simulink library "Lib_General"  (R2023a)
settings: Solver=VariableStepAuto  StartTime=0.0  StopTime=10.0  RelTol=1e-3
settings Model: Creator=62555  LastModifiedBy=62555

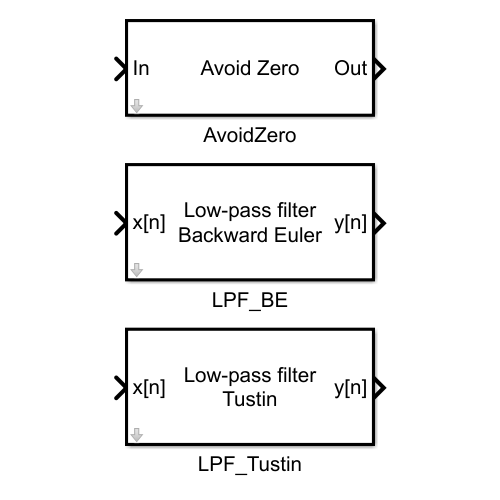
[thumbnail: Simulink's stored preview of the top-level diagram]
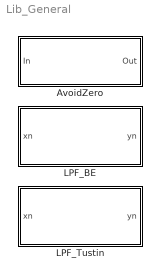
== system Lib_General ==
  AvoidZero : Subsystem  TreatAsAtomicUnit=on  RTWFileName=Lib_General  mask{Min=single(eps)}
      settings: RTWFcnNameOpts=Use subsystem name  RTWFileNameOpts=User specified
      mask Display:
      | disp('Avoid Zero');
      | port_label('input', 1, 'In');
      | port_label('output', 1, 'Out');
  LPF_BE : Subsystem  TreatAsAtomicUnit=on  RTWFileName=Lib_General  mask{fc=1, Ts=1, Initial_condition=0}
      settings: RTWFcnNameOpts=Use subsystem name  RTWFileNameOpts=User specified
      mask Display:
      | disp('Low-pass filter\nBackward Euler');
      | port_label('input', 1, 'x[n]');
      | port_label('output', 1, 'y[n]');
  LPF_Tustin : Subsystem  TreatAsAtomicUnit=on  RTWFileName=Lib_General  mask{fc=1, Ts=1, Initial_condition=0}
      settings: RTWFcnNameOpts=Use subsystem name  RTWFileNameOpts=User specified
      mask Display:
      | disp('Low-pass filter\nTustin');
      | port_label('input', 1, 'x[n]');
      | port_label('output', 1, 'y[n]');

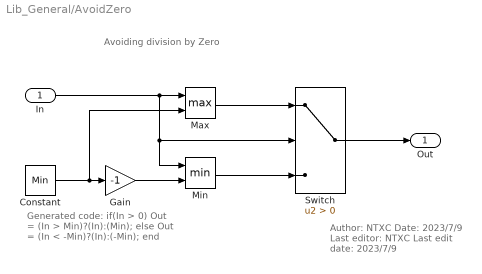
== system Lib_General/AvoidZero ==
  note: Avoiding division by Zero
  note: Generated code:
      |
      | if(In > 0)
      |   Out = (In > Min)?(In):(Min);
      | else
      |   Out = (In < -Min)?(In):(-Min);
      | end
  note: Author: NTXC
      | Date: 2023/7/9
      | Last editor: NTXC
      | Last edit date: 2023/7/9
  In : Inport
  Constant : Constant  Value=Min  OutDataTypeStr=single  SampleTime=-1
  Gain : Gain  Gain=-1
  Max : MinMax  Function=max  Inputs=2
  Min : MinMax  Inputs=2
  Switch : Switch  Criteria=u2 > Threshold  SaturateOnIntegerOverflow=off  InputSameDT=off
  Out : Outport
  wires:
  In/1 -> Min/1, Switch/2, Max/1
  Max/1 -> Switch/1
  Gain/1 -> Min/2
  Min/1 -> Switch/3
  Constant/1 -> Max/2, Gain/1
  Switch/1 -> Out/1

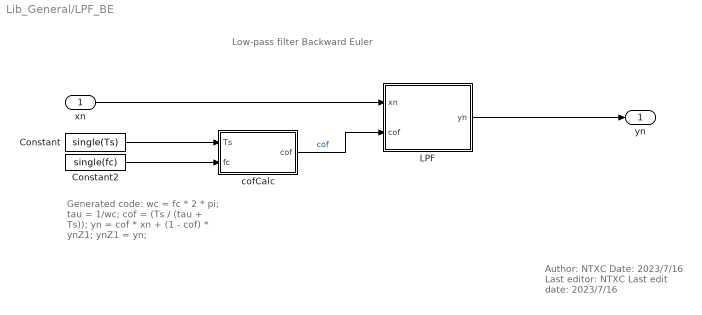
== system Lib_General/LPF_BE ==
  note: Low-pass filter Backward Euler
  note: Author: NTXC
      | Date: 2023/7/16
      | Last editor: NTXC
      | Last edit date: 2023/7/16
  note: Generated code:
      |
      | wc = fc * 2 * pi;
      | tau = 1/wc;
      | cof = (Ts / (tau + Ts));
      |
      | yn = cof * xn + (1 - cof) * ynZ1;
      |
      | ynZ1 = yn;
  xn : Inport
  Constant : Constant  Value=single(Ts)  OutDataTypeStr=single  SampleTime=-1
  Constant2 : Constant  Value=single(fc)  OutDataTypeStr=single  SampleTime=-1
  LPF : Subsystem
  cofCalc : Subsystem
  yn : Outport
  wires:
  Constant/1 -> cofCalc/1(Ts)
  Constant2/1 -> cofCalc/2(fc)
  xn/1 -> LPF/1(xn)
  cofCalc/1(cof) -> LPF/2(cof)  "cof"
  LPF/1(yn) -> yn/1

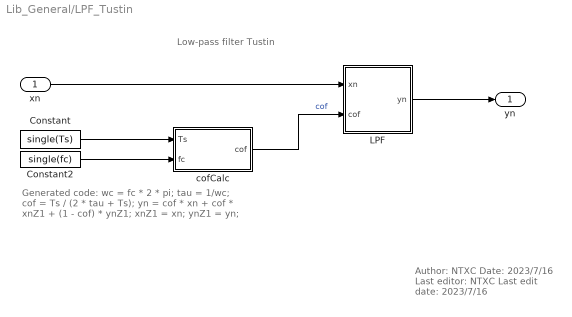
== system Lib_General/LPF_Tustin ==
  note: Author: NTXC
      | Date: 2023/7/16
      | Last editor: NTXC
      | Last edit date: 2023/7/16
  note: Low-pass filter Tustin
  note: Generated code:
      |
      | wc = fc * 2 * pi;
      | tau = 1/wc;
      | cof = Ts / (2 * tau + Ts);
      |
      | yn = cof * xn + cof * xnZ1 + (1 - cof) * ynZ1;
      |
      | xnZ1 = xn;
      | ynZ1 = yn;
  xn : Inport
  Constant : Constant  Value=single(Ts)  OutDataTypeStr=single  SampleTime=-1
  Constant2 : Constant  Value=single(fc)  OutDataTypeStr=single  SampleTime=-1
  LPF : Subsystem
  cofCalc : Subsystem
  yn : Outport
  wires:
  xn/1 -> LPF/1(xn)
  cofCalc/1(cof) -> LPF/2(cof)  "cof"
  LPF/1(yn) -> yn/1
  Constant/1 -> cofCalc/1(Ts)
  Constant2/1 -> cofCalc/2(fc)

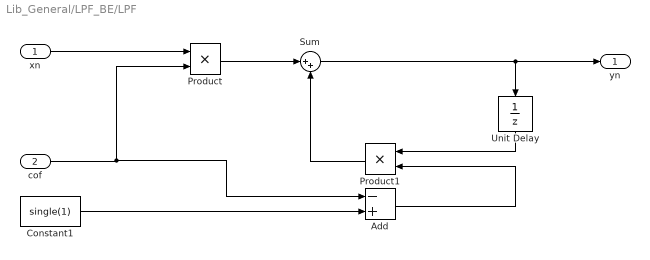
== system Lib_General/LPF_BE/LPF ==
  xn : Inport
  cof : Inport  Port=2
  Add : Sum  Inputs=-+
  Constant1 : Constant  Value=single(1)  OutDataTypeStr=single  SampleTime=-1
  Product : Product
  Product1 : Product
  Sum : Sum  Inputs=|++
  Unit Delay : UnitDelay  InitialCondition=single(Initial_condition)  SampleTime=-1  HasFrameUpgradeWarning=on
  yn : Outport
  wires:
  Add/1 -> Product1/2
  Product1/1 -> Sum/2
  Product/1 -> Sum/1
  Sum/1 -> yn/1, Unit Delay/1
  Unit Delay/1 -> Product1/1
  Constant1/1 -> Add/2
  cof/1 -> Add/1, Product/2
  xn/1 -> Product/1

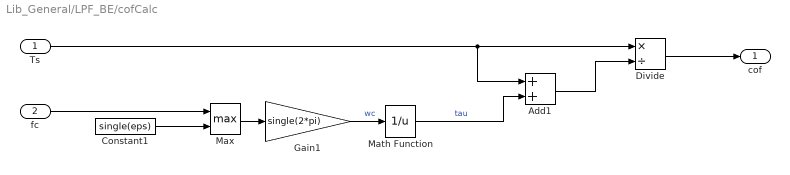
== system Lib_General/LPF_BE/cofCalc ==
  Ts : Inport
  fc : Inport  Port=2
  Add1 : Sum
  Constant1 : Constant  Value=single(eps)  OutDataTypeStr=single  SampleTime=-1
  Divide : Product  Inputs=*/
  Gain1 : Gain  Gain=single(2*pi)
  Math Function : Math  Operator=reciprocal
  Max : MinMax  Function=max  Inputs=2
  cof : Outport
  wires:
  Constant1/1 -> Max/2
  Gain1/1 -> Math Function/1  "wc"
  Max/1 -> Gain1/1
  fc/1 -> Max/1
  Add1/1 -> Divide/2
  Math Function/1 -> Add1/2  "tau"
  Ts/1 -> Add1/1, Divide/1
  Divide/1 -> cof/1

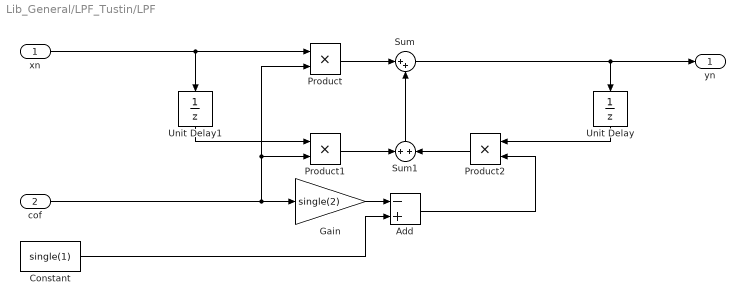
== system Lib_General/LPF_Tustin/LPF ==
  xn : Inport
  cof : Inport  Port=2
  Add : Sum  Inputs=-+
  Constant : Constant  Value=single(1)  OutDataTypeStr=single  SampleTime=-1
  Gain : Gain  Gain=single(2)
  Product : Product
  Product1 : Product
  Product2 : Product
  Sum : Sum  Inputs=|++
  Sum1 : Sum  Inputs=+|+
  Unit Delay : UnitDelay  InitialCondition=single(Initial_condition)  SampleTime=-1  HasFrameUpgradeWarning=on
  Unit Delay1 : UnitDelay  InitialCondition=single(Initial_condition)  SampleTime=-1  HasFrameUpgradeWarning=on
  yn : Outport
  wires:
  Sum/1 -> Unit Delay/1, yn/1
  Unit Delay/1 -> Product2/1
  Product1/1 -> Sum1/1
  xn/1 -> Unit Delay1/1, Product/1
  cof/1 -> Gain/1, Product1/2, Product/2
  Unit Delay1/1 -> Product1/1
  Product/1 -> Sum/1
  Product2/1 -> Sum1/2
  Sum1/1 -> Sum/2
  Gain/1 -> Add/1
  Add/1 -> Product2/2
  Constant/1 -> Add/2

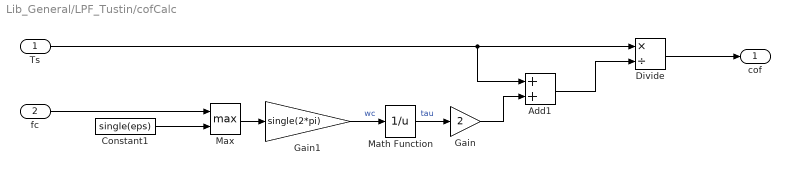
== system Lib_General/LPF_Tustin/cofCalc ==
  Ts : Inport
  fc : Inport  Port=2
  Add1 : Sum
  Constant1 : Constant  Value=single(eps)  OutDataTypeStr=single  SampleTime=-1
  Divide : Product  Inputs=*/
  Gain : Gain  Gain=2
  Gain1 : Gain  Gain=single(2*pi)
  Math Function : Math  Operator=reciprocal
  Max : MinMax  Function=max  Inputs=2
  cof : Outport
  wires:
  Divide/1 -> cof/1
  Ts/1 -> Divide/1, Add1/1
  Math Function/1 -> Gain/1  "tau"
  Gain/1 -> Add1/2
  Add1/1 -> Divide/2
  fc/1 -> Max/1
  Max/1 -> Gain1/1
  Gain1/1 -> Math Function/1  "wc"
  Constant1/1 -> Max/2
